simulink model "MIMO_Case_B_MPC_MHE"  (R2024b)
settings: Solver=ode45  StartTime=0.0  StopTime=p.Tmax  FixedStep=p.Ts  RelTol=1e-3
values from neighbouring files (symbols this model uses):
  iin_ref = 1    [MIMO_Case_B_MPC_MHE_compensator.m]    (also in plotting.m = out.iin.get('r'))
  N = 4    [MIMO_Case_B_MPC_MHE_compensator.m]
  nu = 2    [MHE_estimator.m]    (also in MIMO_Case_B_MPC_MHE_compensator.m; MPC_controller.m)
  nx = 3    [MHE_estimator.m]    (also in MIMO_Case_B_MPC_MHE_compensator.m; MPC_controller.m)
  p = MIMO_Case_B_params()    [MHE_estimator.m]    (also in MIMO_Case_B_MPC_MHE_compensator.m; MPC_controller.m)
  x_0 = [0 ... (first row only)    [MIMO_Case_B_MPC_MHE_compensator.m]
undefined symbols (not defined in the file or in its folder): plecs
settings Model: Creator=rickd  LastModifiedBy=rickd

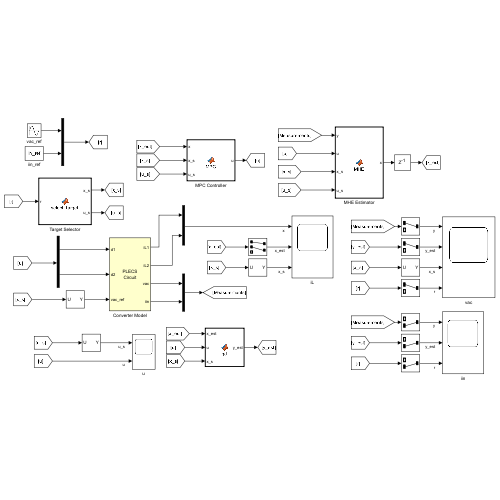
[thumbnail: Simulink's stored preview of the top-level diagram]
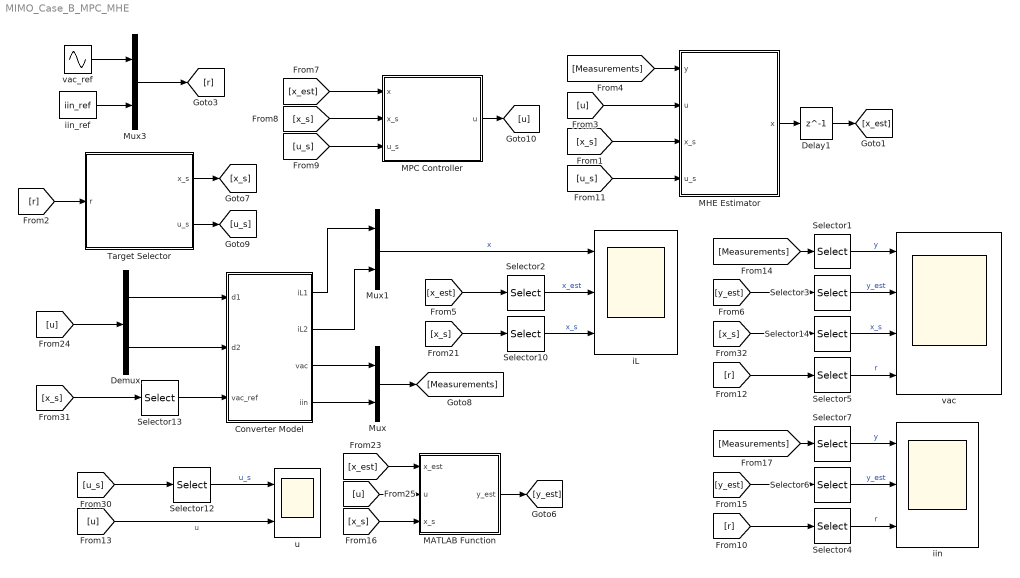
== system MIMO_Case_B_MPC_MHE ==
  Converter Model : Subsystem  LoadFcn=plecs('sl', 200);  InitFcn=plecs('sl', 214);  StartFcn=plecs('sl', 208);  StopFcn=plecs('sl', 209);  mask(PlecsCircuit){PLECSData=<binary blob, 10112 chars, not shown>}
      mask prompts: PLECSData "PLECS Data (Do not delete or modify!)"
      mask init:
      | % PLACE CUSTOM INITIALIZATIONS ABOVE
      | % DO NOT REMOVE
      | plecs('sl', 215);
      | % DO NOT REMOVE
      settings: CopyFcn=plecs('sl', 203);  DeleteFcn=plecs('sl', 205);  UndoDeleteFcn=plecs('sl', 206);  PreSaveFcn=plecs('sl', 211);  PostSaveFcn=plecs('sl', 201);  NameChangeFcn=plecs('sl', 210);  DestroyFcn=plecs('sl', 207);  PreCopyFcn=plecs('sl', 216);  OpenFcn=plecs('sl', 202);  ErrorFcn=plerrorfcn
      mask Help: eval('plecs(''help'', ''qthelp:///creatingacircuit.html'')')
      mask Display: disp('PLECS\nCircuit')
  Delay1 : Delay  DelayLength=1  InitialCondition=x_0  SampleTime=p.Ts
  Demux : Demux  Outputs=2
  MATLAB Function : MATLAB Function  TreatAsAtomicUnit=on  SystemSampleTime=p.Ts
  MHE Estimator : MATLAB Function  TreatAsAtomicUnit=on  SystemSampleTime=p.Ts
  MPC Controller : MATLAB Function  TreatAsAtomicUnit=on  SystemSampleTime=p.Ts
  Mux : Mux  Inputs=ny
  Mux1 : Mux  Inputs=nx-1
  Mux3 : Mux  Inputs=2
  Selector1 : Selector  InputPortWidth=ny  IndexOptions=Index vector (dialog)  Indices=1  OutputSizes=1
  Selector10 : Selector  InputPortWidth=(N+1)*nx  IndexOptions=Index vector (dialog)  Indices=[1:2]  OutputSizes=1
  Selector12 : Selector  InputPortWidth=(N+1)*nu  IndexOptions=Index vector (dialog)  Indices=[1:nu]  OutputSizes=1
  Selector13 : Selector  InputPortWidth=(N+1)*nx  IndexOptions=Index vector (dialog)  Indices=nx  OutputSizes=1
  Selector14 : Selector  InputPortWidth=(N+1)*nx  IndexOptions=Index vector (dialog)  Indices=3  OutputSizes=1
  Selector2 : Selector  InputPortWidth=nx  IndexOptions=Index vector (dialog)  Indices=[1, 2]  OutputSizes=1
  Selector3 : Selector  InputPortWidth=ny  IndexOptions=Index vector (dialog)  Indices=1  OutputSizes=1
  Selector4 : Selector  InputPortWidth=ny  IndexOptions=Index vector (dialog)  Indices=2  OutputSizes=1
  Selector5 : Selector  InputPortWidth=ny  IndexOptions=Index vector (dialog)  Indices=1  OutputSizes=1
  Selector6 : Selector  InputPortWidth=ny  IndexOptions=Index vector (dialog)  Indices=2  OutputSizes=1
  Selector7 : Selector  InputPortWidth=ny  IndexOptions=Index vector (dialog)  Indices=2  OutputSizes=1
  Target Selector : MATLAB Function  TreatAsAtomicUnit=on  SystemSampleTime=p.Ts
  iL : Scope  NumInputPorts=3
  iin : Scope  NumInputPorts=3
  iin_ref : Constant  Value=iin_ref  SampleTime=p.Ts
  u : Scope  NumInputPorts=2
  vac : Scope  NumInputPorts=4
  vac_ref : Sin  Amplitude=p.Vac  Frequency=2*pi*p.fgrid  SampleTime=0
  wires:
  MPC Controller/1(u) -> [u]
  Converter Model/3(vac) -> Mux/1
  Converter Model/1(iL1) -> Mux1/1
  Converter Model/2(iL2) -> Mux1/2
  [x_s] -> MPC Controller/2(x_s)
  [u_s] -> MPC Controller/3(u_s)
  Selector1/1 -> vac/1  "y"
  Selector14/1 -> vac/3  "x_s"
  Selector7/1 -> iin/1  "y"
  [x_s] -> Selector10/1
  Selector10/1 -> iL/3  "x_s"
  Demux/1 -> Converter Model/1(d1)
  Demux/2 -> Converter Model/2(d2)
  [u] -> Demux/1
  [u_s] -> Selector12/1
  Selector12/1 -> u/1  "u_s"
  [x_s] -> Selector13/1
  Selector13/1 -> Converter Model/3(vac_ref)
  [x_s] -> Selector14/1
  [x_s] -> MHE Estimator/3(x_s)
  Selector2/1 -> iL/2  "x_est"
  [x_est] -> Selector2/1
  [y_est] -> Selector3/1
  Selector3/1 -> vac/2  "y_est"
  Mux1/1 -> iL/1  "x"
  [Measurements] -> MHE Estimator/1(y)
  [u] -> MHE Estimator/2(u)
  vac_ref/1 -> Mux3/1
  iin_ref/1 -> Mux3/2
  Mux3/1 -> [r]
  [r] -> Target Selector/1(r)
  Selector4/1 -> iin/3  "r"
  [r] -> Selector4/1
  MHE Estimator/1(x) -> Delay1/1
  Delay1/1 -> [x_est]
  [u_s] -> MHE Estimator/4(u_s)
  Converter Model/4(iin) -> Mux/2
  [r] -> Selector5/1
  Selector5/1 -> vac/4  "r"
  [x_est] -> MPC Controller/1(x)
  Target Selector/1(x_s) -> [x_s]
  Target Selector/2(u_s) -> [u_s]
  Mux/1 -> [Measurements]
  [u] -> u/2  "u"
  MATLAB Function/1(y_est) -> [y_est]
  [x_est] -> MATLAB Function/1(x_est)
  [u] -> MATLAB Function/2(u)
  [x_s] -> MATLAB Function/3(x_s)
  [Measurements] -> Selector1/1
  [y_est] -> Selector6/1
  Selector6/1 -> iin/2  "y_est"
  [Measurements] -> Selector7/1

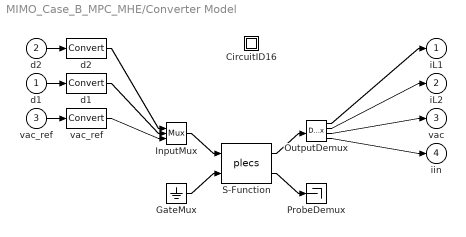
== system MIMO_Case_B_MPC_MHE/Converter Model ==
  d1 : Inport  PortDimensions=1
  d2 : Inport  Port=2  PortDimensions=1
  vac_ref : Inport  Port=3  PortDimensions=1
  " CircuitID16 " : Subsystem
  " GateMux " : Ground
  " InputMux " : Mux  Inputs=[ 1 1 1 ]
  " OutputDemux " : Demux  Outputs=[ 1 1 1 1 ]
  " ProbeDemux " : Terminator
  " S-Function " : S-Function  FunctionName=plecs  SFunctionDeploymentMode=off  EnableBusSupport=off
  " d1 " : DataTypeConversion
  " d2 " : DataTypeConversion
  " vac_ref " : DataTypeConversion
  iL1 : Outport  PortDimensions=1
  iL2 : Outport  Port=2  PortDimensions=1
  vac : Outport  Port=3  PortDimensions=1
  iin : Outport  Port=4  PortDimensions=1
  wires:
  " InputMux "/1 -> " S-Function "/1
  " GateMux "/1 -> " S-Function "/2
  " S-Function "/1 -> " OutputDemux "/1
  " S-Function "/2 -> " ProbeDemux "/1
  d2/1 -> " d2 "/1
  " d2 "/1 -> " InputMux "/1
  d1/1 -> " d1 "/1
  " d1 "/1 -> " InputMux "/2
  vac_ref/1 -> " vac_ref "/1
  " vac_ref "/1 -> " InputMux "/3
  " OutputDemux "/1 -> iL1/1
  " OutputDemux "/2 -> iL2/1
  " OutputDemux "/3 -> vac/1
  " OutputDemux "/4 -> iin/1

== system MIMO_Case_B_MPC_MHE/Converter Model/ CircuitID16  ==

== matlab function MIMO_Case_B_MPC_MHE/Target Selector ==
  data: r input; x_s output; u_s output; mpc parameter
function [x_s, u_s] = select_target(r, mpc)

options = optimoptions('fsolve', 'Algorithm', 'levenberg-marquardt');

p = mpc.p;

N = mpc.N;
nx = mpc.nx;
nu = mpc.nu;

persistent xu_0
if isempty(xu_0), xu_0 = zeros(nx+nu,1); end

persistent sign_cos
if isempty(sign_cos), sign_cos = 1; end
if abs(r(1)) == p.Vac
    sign_cos = sign_cos * (-1);
end

persistent X_S U_S iin_ref_old
if isempty(iin_ref_old), iin_ref_old = 0; end
if (isempty(X_S) && isempty(U_S)) || (iin_ref_old ~= r(2))
    X_S = zeros((N+1)*nx, 1);
    U_S = zeros((N+1)*nu, 1);
    for k=0:N
        vac_ref = r(1) * cos(2*pi*p.fgrid*k*p.Ts) + sign_cos * sqrt(p.Vac^2 - r(1)^2) * sin(2*pi*p.fgrid*k*p.Ts);
    
        fun = @(xu) dynamics_wrapper(xu, [vac_ref; r(2)], p, nx, nu) - [zeros(nx,1); [vac_ref; r(2)]];
    
        sol = fsolve(fun, xu_0, options);

        xu_0 = sol;

        X_S(k*nx+1:(k+1)*nx,1) = sol(1:nx);
        U_S(k*nu+1:(k+1)*nu,1) = sol(nx+1:nx+nu);
    end
else
    vac_ref = r(1) * cos(2*pi*p.fgrid*N*p.Ts) + sign_cos * sqrt(p.Vac^2 - r(1)^2) * sin(2*pi*p.fgrid*N*p.Ts);

    fun = @(xu) dynamics_wrapper(xu, [vac_ref; r(2)], p, nx, nu) - [zeros(nx,1); [vac_ref; r(2)]];
    
    sol = fsolve(fun, xu_0, options);

    xu_0 = sol;
    
    solx = sol(1:nx);
    solu = sol(nx+1:nx+nu);
    
    X_S = [X_S(nx+1:end,1); solx];
    U_S = [U_S(nu+1:end,1); solu];
end

iin_ref_old = r(2);

x_s = X_S;
u_s = U_S;

% Wrapper function to select the appropriate dynamics function
function out = dynamics_wrapper(xu, r, p, nx, nu)
    x = xu(1:nx);
    u = xu(nx+1:nx+nu);

    if r(1) >= 0
        [xdot, y] = MIMO_Case_B_dynamics_SM1(x, u, p);
    else
        [xdot, y] = MIMO_Case_B_dynamics_SM2(x, u, p);
    end

    out = [xdot; y];
end

end

== matlab function MIMO_Case_B_MPC_MHE/MPC Controller ==
  data: x input; x_s input; u_s input; u output; mpc parameter
function u = MPC(x, x_s, u_s, mpc)

coder.extrinsic('fprintf');
options = optimoptions('fmincon', 'Algorithm', 'sqp');

p = mpc.p;
f = @(x, u, x_s) dynamics_wrapper(x, u, x_s, p);
k1 = @(x, u, x_s) f(x, u, x_s);
k2 = @(x, u, x_s) f(x + p.Ts/2*k1(x,u,x_s), u, x_s);
k3 = @(x, u, x_s) f(x + p.Ts/2*k2(x,u,x_s), u, x_s);
k4 = @(x, u, x_s) f(x + p.Ts*k3(x,u,x_s), u, x_s);
fd = @(x, u, x_s) x + p.Ts/6*(k1(x,u,x_s) + 2*k2(x,u,x_s) + 2*k3(x,u,x_s) + k4(x,u,x_s));

N = mpc.N;
nx = mpc.nx;
nu = mpc.nu;

Pf = zeros(nx, nx);
HxN = mpc.Hx;
hxN = mpc.hx;

Hessian = blkdiag(mpc.QX, Pf, mpc.RU);
fun = @(z) 1/2*((z - [x_s; u_s(1:end-nu,1)])' * Hessian * (z - [x_s; u_s(1:end-nu,1)]));
H = blkdiag(kron(eye(N), mpc.Hx), HxN, kron(eye(N), mpc.Hu));
h = [repmat(mpc.hx, N, 1);
     hxN;
     repmat(mpc.hu, N, 1)];
nonlcon = @(z) nlcon(z, fd, x, x_s, nx, nu, N);

persistent z_0
if isempty(z_0), z_0 = mpc.z_0; end
[z, fval, exitflag, ~] = fmincon(fun, z_0, H, h, [], [], [], [], nonlcon, options);
u = z((N+1)*nx+1:(N+1)*nx+nu,1);
z_0 = z;

persistent iter max_fval
if isempty(iter), iter = 0; end
iter = iter + 1;
if isempty(max_fval), max_fval = 0; end
if fval > max_fval && iter > N+1
    max_fval = fval;
end
fprintf('Iteration: %d, ', iter)
fprintf('Cost: %f, ', fval)
fprintf('Worst-case cost: %f, ', max_fval)
fprintf('Exitflag: %f\n', exitflag)

function [c, ceq] = nlcon(z, f, x, x_s, nx, nu, N)
    c = [];
    c1 = zeros(N*nx, 1); % Preallocate
    for i = 1:N
        c1((i-1)*nx+1:i*nx,1) = z(i*nx+1:(i+1)*nx,1) - f(z((i-1)*nx+1:i*nx,1), z((N+1)*nx+(i-1)*nu+1:(N+1)*nx+i*nu,1), x_s((i-1)*nx+1:i*nx,1));
    end
    ceq = [z(1:nx,1) - x; c1]; % Equality constraints
end

% Wrapper function to select the appropriate dynamics function
function xdot = dynamics_wrapper(x, u, x_s, p)
    if x_s(3) >= 0
        [xdot, ~] = MIMO_Case_B_dynamics_SM1(x, u, p);
    else
        [xdot, ~] = MIMO_Case_B_dynamics_SM2(x, u, p);
    end
end

end

== matlab function MIMO_Case_B_MPC_MHE/MHE Estimator ==
  data: y input; u input; x_s input; u_s input; x output; mhe parameter
function x = MHE(y, u, x_s, u_s, mhe)

options = optimoptions('fmincon', 'Algorithm', 'sqp');

p = mhe.p;
f = @(x, u, x_s) dynamics_wrapper(x, u, x_s, p);
k1 = @(x, u, x_s) f(x, u, x_s);
k2 = @(x, u, x_s) f(x + p.Ts/2*k1(x,u,x_s), u, x_s);
k3 = @(x, u, x_s) f(x + p.Ts/2*k2(x,u,x_s), u, x_s);
k4 = @(x, u, x_s) f(x + p.Ts*k3(x,u,x_s), u, x_s);
fd = @(x, u, x_s) x + p.Ts/6*(k1(x,u,x_s) + 2*k2(x,u,x_s) + 2*k3(x,u,x_s) + k4(x,u,x_s));
gd = @(x, u, x_s) output_wrapper(x, u, x_s, p);

N = mhe.N;
nx = mhe.nx;
nu = mhe.nu;
ny = mhe.ny;

persistent x_bar P P_ekf
if isempty(x_bar), x_bar = zeros(N*(nx), 1); end
if isempty(P), P = repmat(eye(nx), N, 1); end
if isempty(P_ekf), P_ekf = mhe.Q; end

persistent Y  U  Xs
if isempty(Y), Y = zeros(N*ny, 1); end
if isempty(U), U = zeros(N*nu, 1); end
if isempty(Xs), Xs = zeros(N*nx, 1); end
Y = [Y(ny+1:end,1); y];
U = [U(nu+1:end,1); u];
Xs = [Xs(nx+1:end,1); x_s(1:nx,1)];

fun = @(z) 1/2*(z((N+1)*nx+1:end,1)' * mhe.QW * z((N+1)*nx+1:end,1) + (Y - gdN(gd, z(1:N*nx,1), U, Xs, N, nx, nu, ny))' * mhe.RV * (Y - gdN(gd, z(1:N*nx,1), U, Xs, N, nx, nu, ny)) + (x_bar(1:nx,1) - z(1:nx,1))' * (P(1:nx,:) \ (x_bar(1:nx,1) - z(1:nx,1))));
nonlcon = @(z) nlcon(z, U, fd, N, nx, nu, Xs);
persistent z_0
if isempty(z_0), z_0 = mhe.z_0; end
z = fmincon(fun, z_0, [], [], [], [], [], [], nonlcon, options);
x = z(N*nx+1:(N+1)*nx,1);
z_0 = z;
x_bar = [x_bar(nx+1:end,1); x];

% update EKF
if x_s(3) >= 0
    A = A1(x_s(1:nx,1), u_s(1:nu,1));
    C = C1(x_s(1:nx,1), u_s(1:nu,1));
else
    A = A2(x_s(1:nx,1), u_s(1:nu,1));
    C = C2(x_s(1:nx,1), u_s(1:nu,1));
end
% Measurement update
L = ((C * P_ekf * C' + mhe.R)\(C * P_ekf))';
P_ekf = P_ekf - L * C * P_ekf;
% Time update
P_ekf = A * P_ekf * A' + mhe.Q;
P = [P(nx+1:end,:); P_ekf];

function [c, ceq] = nlcon(z, u, f, N, nx, nu, x_s)
    c = []; % No inequality constraints
    c1 = zeros(N*nx, 1); % Preallocate
    for i = 1:N
        c1((i-1)*nx+1:i*nx,1) = z(i*nx+1:(i+1)*nx,1) - f(z((i-1)*nx+1:i*nx,1), u((i-1)*nu+1:i*nu,1), x_s((i-1)*nx+1:i*nx,1)) - z((N+1)*nx+(i-1)*nx+1:(N+1)*nx+i*nx,1); % x_k+1 = f(x_k, u_k) + w_k
    end
    ceq = c1;
end

% Wrapper function to select the appropriate dynamics function
function xdot = dynamics_wrapper(x, u, x_s, p)
    if x_s(3) >= 0
        [xdot, ~] = MIMO_Case_B_dynamics_SM1(x, u, p);
    else
        [xdot, ~] = MIMO_Case_B_dynamics_SM2(x, u, p);
    end
end

function y = output_wrapper(x, u, x_s, p)
    if x_s(3) >= 0
        [~, y] = MIMO_Case_B_dynamics_SM1(x, u, p);
    else
        [~, y] = MIMO_Case_B_dynamics_SM2(x, u, p);
    end
end

function out = gdN(g, x, u, x_s, N, nx, nu, ny)
    % Initialize output
    out = zeros(N*ny, 1);

    % Loop through each time step
    for i = 1:N
        % Extract single time step state and control input
        x_i = x((i-1)*nx + (1:nx)); % nx-by-1
        u_i = u((i-1)*nu + (1:nu)); % nu-by-1
        x_si = x_s((i-1)*nx + (1:nx)); % nx-by-1

        % Compute gd for this step and store result
        out((i-1)*ny + (1:ny)) = g(x_i, u_i, x_si);
    end
end

end

== matlab function MIMO_Case_B_MPC_MHE/MATLAB Function ==
  data: x_est input; u input; y_est output; x_s input; p parameter
function y_est = gd(x_est, u, x_s, p)

y_est = output_wrapper(x_est, u, x_s, p);

function y = output_wrapper(x, u, x_s, p)
    if x_s(3) >= 0
        [~, y] = MIMO_Case_B_dynamics_SM1(x, u, p);
    else
        [~, y] = MIMO_Case_B_dynamics_SM2(x, u, p);
    end
end

end
